simulink model "BCM_C1A_CombiSwitch_9"  (R2018b)
settings: Solver=FixedStepDiscrete  StartTime=0.0  StopTime=10.0  FixedStep=0.01  RelTol=1e-3
undefined symbols (not defined in the file or in its folder): TYP_CSW_INT_POSITION, TYP_EXT_LIGHTS, TYP_FRONT_WIPER, TYP_LIGHTING_CSW, TYP_REAR_WIPER, TYP_VEHICLE_STATE
libraries: Renault_Library x80, library_BCM x2
(part 3 of 3)

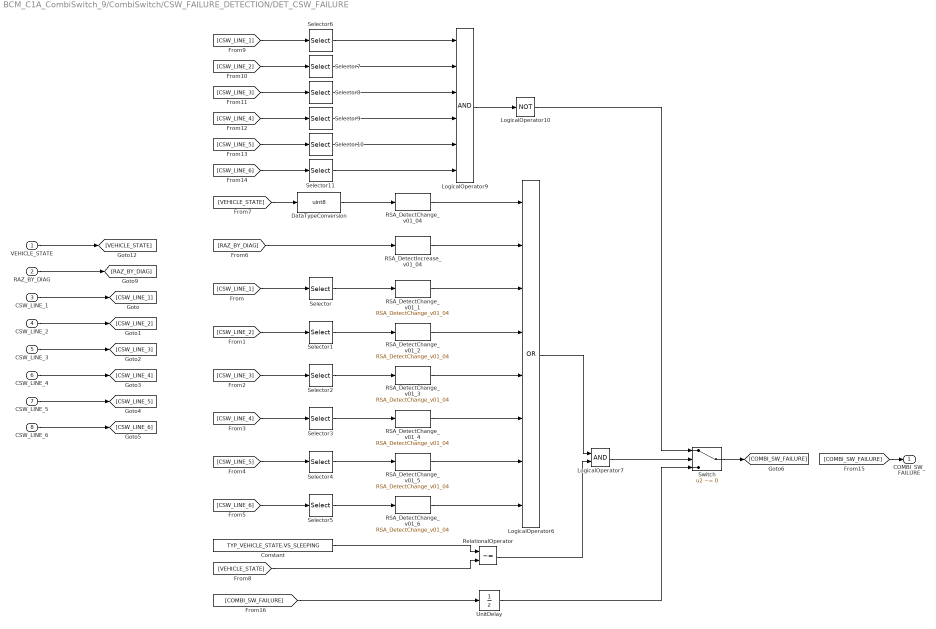
== system BCM_C1A_CombiSwitch_9/CombiSwitch/CSW_FAILURE_DETECTION/DET_CSW_FAILURE ==
  VEHICLE_STATE : Inport  OutDataTypeStr=Enum: TYP_VEHICLE_STATE
      settings: AttributesFormatString=Type : %<OutDataTypeStr>
  RAZ_BY_DIAG : Inport  Port=2  OutDataTypeStr=boolean
      settings: AttributesFormatString=Type : %<OutDataTypeStr>
  CSW_LINE_1 : Inport  Port=3  OutDataTypeStr=boolean  PortDimensions=6
      settings: AttributesFormatString=Type : %<OutDataTypeStr>
  CSW_LINE_2 : Inport  Port=4  OutDataTypeStr=boolean  PortDimensions=6
      settings: AttributesFormatString=Type : %<OutDataTypeStr>
  CSW_LINE_3 : Inport  Port=5  OutDataTypeStr=boolean  PortDimensions=6
      settings: AttributesFormatString=Type : %<OutDataTypeStr>
  CSW_LINE_4 : Inport  Port=6  OutDataTypeStr=boolean  PortDimensions=6
      settings: AttributesFormatString=Type : %<OutDataTypeStr>
  CSW_LINE_5 : Inport  Port=7  OutDataTypeStr=boolean  PortDimensions=6
      settings: AttributesFormatString=Type : %<OutDataTypeStr>
  CSW_LINE_6 : Inport  Port=8  OutDataTypeStr=boolean  PortDimensions=6
      settings: AttributesFormatString=Type : %<OutDataTypeStr>
  Constant : Constant  Value=TYP_VEHICLE_STATE.VS_SLEEPING  OutDataTypeStr=Enum: TYP_VEHICLE_STATE  SampleTime=-1
  DataTypeConversion : DataTypeConversion  OutDataTypeStr=uint8  RndMeth=Zero
      settings: AttributesFormatString=Saturation:%<SaturateOnIntegerOverflow>
  LogicalOperator10 : Logic  Operator=NOT  Inputs=1  OutDataTypeStr=boolean
  LogicalOperator6 : Logic  Operator=OR  Inputs=8  OutDataTypeStr=boolean
  LogicalOperator7 : Logic  OutDataTypeStr=boolean
  LogicalOperator9 : Logic  Inputs=6  OutDataTypeStr=boolean
  RSA_DetectChange_v01_04 : Renault_Library/Complex blocks/Logic & Bit Operations/RSA_DetectChange_v01_04  Tag=[LIB]  chkini=on  vinit=false
      settings: AttributesFormatString=%<MaskType> : Ver : 01.04\nCompare the Input with Initial Value = %<chkini>\nInitial Value : = %<vinit>
  RSA_DetectChange_v01_{1..6} (6 alike) : Renault_Library/Complex blocks/Logic & Bit Operations/RSA_DetectChange_v01_04  Tag=[LIB]  chkini=on  vinit=false
      settings: AttributesFormatString=%<MaskType> : Ver : 01.04\nCompare the Input with Initial Value = %<chkini>\nInitial Value : = %<vinit>
  RSA_DetectIncrease_v01_04 : Renault_Library/Complex blocks/Logic & Bit Operations/RSA_DetectIncrease_v01_04  Tag=[LIB]  chkini=on  vinit=false
      settings: AttributesFormatString=%<MaskType> : Ver : 01.04\nCompare the Input with Initial Value = %<chkini>\nInitial Value : = %<vinit>
  RelationalOperator : RelationalOperator  Operator=~=  OutDataTypeStr=boolean  RndMeth=Nearest  InputSameDT=on
  Selector : Selector  IndexMode=Zero-based  InputPortWidth=6  IndexOptions=Index vector (dialog)  Indices=[0]  OutputSizes=1
  Selector1 : Selector  IndexMode=Zero-based  InputPortWidth=6  IndexOptions=Index vector (dialog)  Indices=[1]  OutputSizes=1
  Selector10 : Selector  IndexMode=Zero-based  InputPortWidth=6  IndexOptions=Index vector (dialog)  Indices=[4]  OutputSizes=1
  Selector11 : Selector  IndexMode=Zero-based  InputPortWidth=6  IndexOptions=Index vector (dialog)  Indices=[5]  OutputSizes=1
  Selector2 : Selector  IndexMode=Zero-based  InputPortWidth=6  IndexOptions=Index vector (dialog)  Indices=[2]  OutputSizes=1
  Selector3 : Selector  IndexMode=Zero-based  InputPortWidth=6  IndexOptions=Index vector (dialog)  Indices=[3]  OutputSizes=1
  Selector4 : Selector  IndexMode=Zero-based  InputPortWidth=6  IndexOptions=Index vector (dialog)  Indices=[4]  OutputSizes=1
  Selector5 : Selector  IndexMode=Zero-based  InputPortWidth=6  IndexOptions=Index vector (dialog)  Indices=[5]  OutputSizes=1
  Selector6 : Selector  IndexMode=Zero-based  InputPortWidth=6  IndexOptions=Index vector (dialog)  Indices=[0]  OutputSizes=1
  Selector7 : Selector  IndexMode=Zero-based  InputPortWidth=6  IndexOptions=Index vector (dialog)  Indices=[1]  OutputSizes=1
  Selector8 : Selector  IndexMode=Zero-based  InputPortWidth=6  IndexOptions=Index vector (dialog)  Indices=[2]  OutputSizes=1
  Selector9 : Selector  IndexMode=Zero-based  InputPortWidth=6  IndexOptions=Index vector (dialog)  Indices=[3]  OutputSizes=1
  Switch : Switch  Criteria=u2 ~= 0  RndMeth=Zero  InputSameDT=on
      settings: AttributesFormatString=Criteria=%<Criteria>
  UnitDelay : UnitDelay  InitialCondition=false  SampleTime=-1
      settings: AttributesFormatString=IC = %<X0>
  COMBI_SW_FAILURE : Outport  OutDataTypeStr=boolean
      settings: AttributesFormatString=Type : %<OutDataTypeStr>\nInit :%<InitialOutput>
  wires:
  LogicalOperator9/1 -> LogicalOperator10/1
  Selector6/1 -> LogicalOperator9/1
  Selector8/1 -> LogicalOperator9/3
  Selector9/1 -> LogicalOperator9/4
  Selector10/1 -> LogicalOperator9/5
  Selector11/1 -> LogicalOperator9/6
  Selector7/1 -> LogicalOperator9/2
  [CSW_LINE_6] -> Selector11/1
  [CSW_LINE_5] -> Selector10/1
  [CSW_LINE_4] -> Selector9/1
  [CSW_LINE_3] -> Selector8/1
  [CSW_LINE_2] -> Selector7/1
  [CSW_LINE_1] -> Selector6/1
  LogicalOperator6/1 -> LogicalOperator7/1
  RelationalOperator/1 -> LogicalOperator7/2
  [VEHICLE_STATE] -> RelationalOperator/2
  Constant/1 -> RelationalOperator/1
  [RAZ_BY_DIAG] -> RSA_DetectIncrease_v01_04/1
  DataTypeConversion/1 -> RSA_DetectChange_v01_04/1
  [VEHICLE_STATE] -> DataTypeConversion/1
  Selector2/1 -> RSA_DetectChange_v01_3/1
  Selector3/1 -> RSA_DetectChange_v01_4/1
  Selector4/1 -> RSA_DetectChange_v01_5/1
  Selector5/1 -> RSA_DetectChange_v01_6/1
  Selector1/1 -> RSA_DetectChange_v01_2/1
  Selector/1 -> RSA_DetectChange_v01_1/1
  [CSW_LINE_6] -> Selector5/1
  [CSW_LINE_5] -> Selector4/1
  [CSW_LINE_4] -> Selector3/1
  [CSW_LINE_3] -> Selector2/1
  [CSW_LINE_2] -> Selector1/1
  [CSW_LINE_1] -> Selector/1
  CSW_LINE_6/1 -> [CSW_LINE_6]
  CSW_LINE_5/1 -> [CSW_LINE_5]
  CSW_LINE_4/1 -> [CSW_LINE_4]
  CSW_LINE_3/1 -> [CSW_LINE_3]
  CSW_LINE_2/1 -> [CSW_LINE_2]
  CSW_LINE_1/1 -> [CSW_LINE_1]
  RAZ_BY_DIAG/1 -> [RAZ_BY_DIAG]
  VEHICLE_STATE/1 -> [VEHICLE_STATE]
  LogicalOperator7/1 -> Switch/2
  LogicalOperator10/1 -> Switch/1
  Switch/1 -> [COMBI_SW_FAILURE]
  [COMBI_SW_FAILURE] -> UnitDelay/1
  [COMBI_SW_FAILURE] -> COMBI_SW_FAILURE/1
  UnitDelay/1 -> Switch/3
  RSA_DetectChange_v01_6/1 -> LogicalOperator6/8
  RSA_DetectChange_v01_5/1 -> LogicalOperator6/7
  RSA_DetectChange_v01_4/1 -> LogicalOperator6/6
  RSA_DetectChange_v01_3/1 -> LogicalOperator6/5
  RSA_DetectChange_v01_2/1 -> LogicalOperator6/4
  RSA_DetectChange_v01_1/1 -> LogicalOperator6/3
  RSA_DetectIncrease_v01_04/1 -> LogicalOperator6/2
  RSA_DetectChange_v01_04/1 -> LogicalOperator6/1

== system BCM_C1A_CombiSwitch_9/CombiSwitch/LIGHTING_FAILURE_DETECTION/DET_LIGHTING_FAILURE_3_POSITIONS ==
  VEHICLE_STATE : Inport  OutDataTypeStr=Enum: TYP_VEHICLE_STATE
      settings: AttributesFormatString=Type : %<OutDataTypeStr>
  RAZ_BY_DIAG : Inport  Port=2  OutDataTypeStr=boolean
      settings: AttributesFormatString=Type : %<OutDataTypeStr>
  CSW_LINE_2 : Inport  Port=3  OutDataTypeStr=boolean  PortDimensions=6
      settings: AttributesFormatString=Type : %<OutDataTypeStr>
  CSW_LINE_4 : Inport  Port=4  OutDataTypeStr=boolean  PortDimensions=6
      settings: AttributesFormatString=Type : %<OutDataTypeStr>
  Enable : EnablePort  StatesWhenEnabling=reset
      settings: AttributesFormatString=State : %<StatesWhenEnabling>
  Constant : Constant  Value=TYP_VEHICLE_STATE.VS_SLEEPING  OutDataTypeStr=Enum: TYP_VEHICLE_STATE  SampleTime=-1
  DataTypeConversion : DataTypeConversion  OutDataTypeStr=uint8  RndMeth=Zero
      settings: AttributesFormatString=Saturation:%<SaturateOnIntegerOverflow>
  LogicalOperator10 : Logic  Operator=NOT  Inputs=1  OutDataTypeStr=boolean
  LogicalOperator6 : Logic  Operator=OR  Inputs=5  OutDataTypeStr=boolean
  LogicalOperator7 : Logic  OutDataTypeStr=boolean
  LogicalOperator8 : Logic  Operator=OR  Inputs=3  OutDataTypeStr=boolean
  RSA_DetectChange_v01_04 : Renault_Library/Complex blocks/Logic & Bit Operations/RSA_DetectChange_v01_04  Tag=[LIB]  chkini=on  vinit=false
      settings: AttributesFormatString=%<MaskType> : Ver : 01.04\nCompare the Input with Initial Value = %<chkini>\nInitial Value : = %<vinit>
  RSA_DetectChange_v01_2 : Renault_Library/Complex blocks/Logic & Bit Operations/RSA_DetectChange_v01_04  Tag=[LIB]  chkini=on  vinit=false
      settings: AttributesFormatString=%<MaskType> : Ver : 01.04\nCompare the Input with Initial Value = %<chkini>\nInitial Value : = %<vinit>
  RSA_DetectChange_v01_4 : Renault_Library/Complex blocks/Logic & Bit Operations/RSA_DetectChange_v01_04  Tag=[LIB]  chkini=on  vinit=false
      settings: AttributesFormatString=%<MaskType> : Ver : 01.04\nCompare the Input with Initial Value = %<chkini>\nInitial Value : = %<vinit>
  RSA_DetectChange_v01_5 : Renault_Library/Complex blocks/Logic & Bit Operations/RSA_DetectChange_v01_04  Tag=[LIB]  chkini=on  vinit=false
      settings: AttributesFormatString=%<MaskType> : Ver : 01.04\nCompare the Input with Initial Value = %<chkini>\nInitial Value : = %<vinit>
  RSA_DetectIncrease_v01_04 : Renault_Library/Complex blocks/Logic & Bit Operations/RSA_DetectIncrease_v01_04  Tag=[LIB]  chkini=on  vinit=false
      settings: AttributesFormatString=%<MaskType> : Ver : 01.04\nCompare the Input with Initial Value = %<chkini>\nInitial Value : = %<vinit>
  RelationalOperator : RelationalOperator  Operator=~=  OutDataTypeStr=boolean  RndMeth=Nearest  InputSameDT=on
  Selector : Selector  IndexMode=Zero-based  InputPortWidth=6  IndexOptions=Index vector (dialog)  Indices=[2]  OutputSizes=1
  Selector{2..3,6..7} (4 alike) : Selector  IndexMode=Zero-based  InputPortWidth=6  IndexOptions=Index vector (dialog)  Indices=[4]  OutputSizes=1
  Selector4 : Selector  IndexMode=Zero-based  InputPortWidth=6  IndexOptions=Index vector (dialog)  Indices=[2]  OutputSizes=1
  Switch : Switch  Criteria=u2 ~= 0  RndMeth=Zero  InputSameDT=on
      settings: AttributesFormatString=Criteria=%<Criteria>
  UnitDelay : UnitDelay  InitialCondition=false  SampleTime=-1
      settings: AttributesFormatString=IC = %<X0>
  COMBI_SW_LIGHTING_FAILURE_3_POS : Outport  OutDataTypeStr=boolean  OutputWhenDisabled=reset  InitialOutput=false
      settings: AttributesFormatString=Type : %<OutDataTypeStr>\nInit :%<InitialOutput>
  wires:
  VEHICLE_STATE/1 -> [VEHICLE_STATE]
  RAZ_BY_DIAG/1 -> [RAZ_BY_DIAG]
  CSW_LINE_2/1 -> [CSW_LINE_2]
  CSW_LINE_4/1 -> [CSW_LINE_4]
  [CSW_LINE_2] -> Selector/1
  [CSW_LINE_2] -> Selector2/1
  [CSW_LINE_4] -> Selector3/1
  Selector/1 -> RSA_DetectChange_v01_2/1
  Selector3/1 -> RSA_DetectChange_v01_5/1
  Selector2/1 -> RSA_DetectChange_v01_4/1
  [VEHICLE_STATE] -> DataTypeConversion/1
  DataTypeConversion/1 -> RSA_DetectChange_v01_04/1
  [RAZ_BY_DIAG] -> RSA_DetectIncrease_v01_04/1
  RSA_DetectChange_v01_04/1 -> LogicalOperator6/1
  Constant/1 -> RelationalOperator/1
  [VEHICLE_STATE] -> RelationalOperator/2
  RelationalOperator/1 -> LogicalOperator7/2
  LogicalOperator6/1 -> LogicalOperator7/1
  LogicalOperator7/1 -> Switch/2
  Selector4/1 -> LogicalOperator8/1
  Selector6/1 -> LogicalOperator8/2
  LogicalOperator8/1 -> LogicalOperator10/1
  LogicalOperator10/1 -> Switch/1
  [COMBI_SW_LIGHTING_FAILURE_3_POS] -> UnitDelay/1
  UnitDelay/1 -> Switch/3
  [CSW_LINE_2] -> Selector4/1
  [CSW_LINE_2] -> Selector6/1
  [CSW_LINE_4] -> Selector7/1
  Selector7/1 -> LogicalOperator8/3
  Switch/1 -> COMBI_SW_LIGHTING_FAILURE_3_POS/1, [COMBI_SW_LIGHTING_FAILURE_3_POS]
  RSA_DetectIncrease_v01_04/1 -> LogicalOperator6/2
  RSA_DetectChange_v01_2/1 -> LogicalOperator6/3
  RSA_DetectChange_v01_4/1 -> LogicalOperator6/4
  RSA_DetectChange_v01_5/1 -> LogicalOperator6/5

== system BCM_C1A_CombiSwitch_9/CombiSwitch/LIGHTING_FAILURE_DETECTION/DET_LIGHTING_FAILURE_4_POSITIONS ==
  VEHICLE_STATE : Inport  OutDataTypeStr=Enum: TYP_VEHICLE_STATE
      settings: AttributesFormatString=Type : %<OutDataTypeStr>
  RAZ_BY_DIAG : Inport  Port=2  OutDataTypeStr=boolean
      settings: AttributesFormatString=Type : %<OutDataTypeStr>
  CSW_LINE_2 : Inport  Port=3  OutDataTypeStr=boolean  PortDimensions=6
      settings: AttributesFormatString=Type : %<OutDataTypeStr>
  CSW_LINE_4 : Inport  Port=4  OutDataTypeStr=boolean  PortDimensions=6
      settings: AttributesFormatString=Type : %<OutDataTypeStr>
  Enable : EnablePort  StatesWhenEnabling=reset
      settings: AttributesFormatString=State : %<StatesWhenEnabling>
  Constant : Constant  Value=TYP_VEHICLE_STATE.VS_SLEEPING  OutDataTypeStr=Enum: TYP_VEHICLE_STATE  SampleTime=-1
  DataTypeConversion : DataTypeConversion  OutDataTypeStr=uint8  RndMeth=Zero
      settings: AttributesFormatString=Saturation:%<SaturateOnIntegerOverflow>
  LogicalOperator10 : Logic  Operator=NOT  Inputs=1  OutDataTypeStr=boolean
  LogicalOperator6 : Logic  Operator=OR  Inputs=6  OutDataTypeStr=boolean
  LogicalOperator7 : Logic  OutDataTypeStr=boolean
  LogicalOperator8 : Logic  Operator=OR  Inputs=4  OutDataTypeStr=boolean
  RSA_DetectChange_v01_04 : Renault_Library/Complex blocks/Logic & Bit Operations/RSA_DetectChange_v01_04  Tag=[LIB]  chkini=on  vinit=false
      settings: AttributesFormatString=%<MaskType> : Ver : 01.04\nCompare the Input with Initial Value = %<chkini>\nInitial Value : = %<vinit>
  RSA_DetectChange_v01_{2..5} (4 alike) : Renault_Library/Complex blocks/Logic & Bit Operations/RSA_DetectChange_v01_04  Tag=[LIB]  chkini=on  vinit=false
      settings: AttributesFormatString=%<MaskType> : Ver : 01.04\nCompare the Input with Initial Value = %<chkini>\nInitial Value : = %<vinit>
  RSA_DetectIncrease_v01_04 : Renault_Library/Complex blocks/Logic & Bit Operations/RSA_DetectIncrease_v01_04  Tag=[LIB]  chkini=on  vinit=false
      settings: AttributesFormatString=%<MaskType> : Ver : 01.04\nCompare the Input with Initial Value = %<chkini>\nInitial Value : = %<vinit>
  RelationalOperator : RelationalOperator  Operator=~=  OutDataTypeStr=boolean  RndMeth=Nearest  InputSameDT=on
  Selector : Selector  IndexMode=Zero-based  InputPortWidth=6  IndexOptions=Index vector (dialog)  Indices=[2]  OutputSizes=1
  Selector1 : Selector  IndexMode=Zero-based  InputPortWidth=6  IndexOptions=Index vector (dialog)  Indices=[3]  OutputSizes=1
  Selector{2..3,6..7} (4 alike) : Selector  IndexMode=Zero-based  InputPortWidth=6  IndexOptions=Index vector (dialog)  Indices=[4]  OutputSizes=1
  Selector4 : Selector  IndexMode=Zero-based  InputPortWidth=6  IndexOptions=Index vector (dialog)  Indices=[2]  OutputSizes=1
  Selector5 : Selector  IndexMode=Zero-based  InputPortWidth=6  IndexOptions=Index vector (dialog)  Indices=[3]  OutputSizes=1
  Switch : Switch  Criteria=u2 ~= 0  RndMeth=Zero  InputSameDT=on
      settings: AttributesFormatString=Criteria=%<Criteria>
  UnitDelay : UnitDelay  InitialCondition=false  SampleTime=-1
      settings: AttributesFormatString=IC = %<X0>
  COMBI_SW_LIGHTING_FAILURE_4_POS : Outport  OutDataTypeStr=boolean  OutputWhenDisabled=reset  InitialOutput=false
      settings: AttributesFormatString=Type : %<OutDataTypeStr>\nInit :%<InitialOutput>
  wires:
  Switch/1 -> [COMBI_SW_LIGHTING_FAILURE_4_POS], COMBI_SW_LIGHTING_FAILURE_4_POS/1
  [CSW_LINE_4] -> Selector7/1
  [CSW_LINE_2] -> Selector6/1
  [CSW_LINE_2] -> Selector5/1
  [CSW_LINE_2] -> Selector4/1
  UnitDelay/1 -> Switch/3
  [COMBI_SW_LIGHTING_FAILURE_4_POS] -> UnitDelay/1
  LogicalOperator10/1 -> Switch/1
  LogicalOperator8/1 -> LogicalOperator10/1
  Selector5/1 -> LogicalOperator8/2
  Selector4/1 -> LogicalOperator8/1
  LogicalOperator7/1 -> Switch/2
  LogicalOperator6/1 -> LogicalOperator7/1
  RelationalOperator/1 -> LogicalOperator7/2
  [VEHICLE_STATE] -> RelationalOperator/2
  Constant/1 -> RelationalOperator/1
  RSA_DetectChange_v01_04/1 -> LogicalOperator6/1
  RSA_DetectIncrease_v01_04/1 -> LogicalOperator6/2
  [RAZ_BY_DIAG] -> RSA_DetectIncrease_v01_04/1
  DataTypeConversion/1 -> RSA_DetectChange_v01_04/1
  [VEHICLE_STATE] -> DataTypeConversion/1
  RSA_DetectChange_v01_5/1 -> LogicalOperator6/6
  RSA_DetectChange_v01_4/1 -> LogicalOperator6/5
  RSA_DetectChange_v01_3/1 -> LogicalOperator6/4
  RSA_DetectChange_v01_2/1 -> LogicalOperator6/3
  Selector2/1 -> RSA_DetectChange_v01_4/1
  Selector3/1 -> RSA_DetectChange_v01_5/1
  Selector1/1 -> RSA_DetectChange_v01_3/1
  Selector/1 -> RSA_DetectChange_v01_2/1
  [CSW_LINE_4] -> Selector3/1
  [CSW_LINE_2] -> Selector2/1
  [CSW_LINE_2] -> Selector1/1
  [CSW_LINE_2] -> Selector/1
  CSW_LINE_4/1 -> [CSW_LINE_4]
  CSW_LINE_2/1 -> [CSW_LINE_2]
  RAZ_BY_DIAG/1 -> [RAZ_BY_DIAG]
  VEHICLE_STATE/1 -> [VEHICLE_STATE]
  Selector6/1 -> LogicalOperator8/3
  Selector7/1 -> LogicalOperator8/4

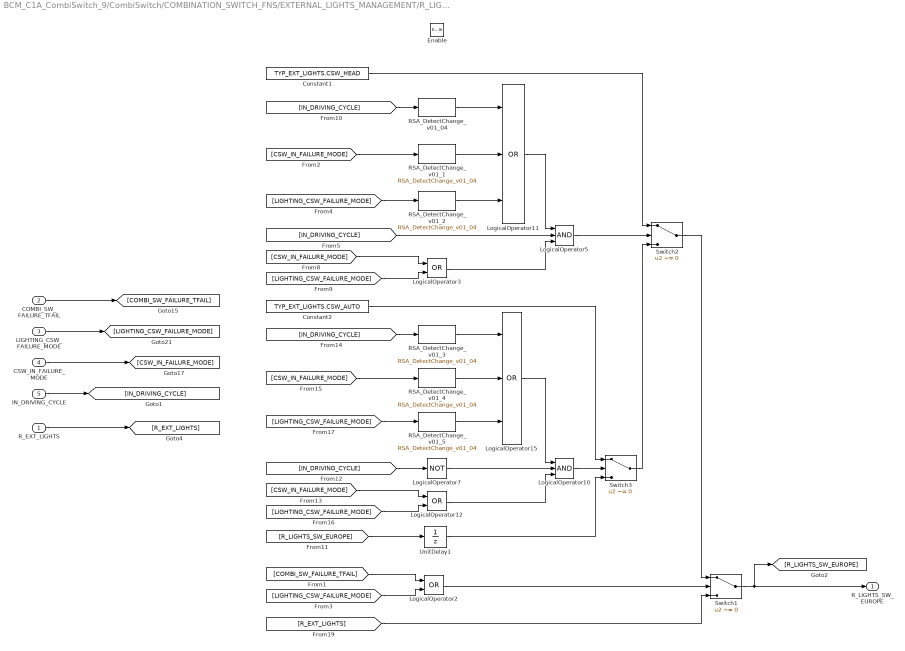
== system BCM_C1A_CombiSwitch_9/CombiSwitch/COMBINATION_SWITCH_FNS/EXTERNAL_LIGHTS_MANAGEMENT/R_LIGHT_SW_EUROPE ==
  R_EXT_LIGHTS : Inport  OutDataTypeStr=Enum: TYP_EXT_LIGHTS
      settings: AttributesFormatString=Type : %<OutDataTypeStr>
  COMBI_SW_FAILURE_TFAIL : Inport  Port=2  OutDataTypeStr=boolean
      settings: AttributesFormatString=Type : %<OutDataTypeStr>
  LIGHTING_CSW_FAILURE_MODE : Inport  Port=3  OutDataTypeStr=boolean
      settings: AttributesFormatString=Type : %<OutDataTypeStr>
  CSW_IN_FAILURE_MODE : Inport  Port=4  OutDataTypeStr=boolean
      settings: AttributesFormatString=Type : %<OutDataTypeStr>
  IN_DRIVING_CYCLE : Inport  Port=5  OutDataTypeStr=boolean
      settings: AttributesFormatString=Type : %<OutDataTypeStr>
  Enable : EnablePort  StatesWhenEnabling=reset
      settings: AttributesFormatString=State : %<StatesWhenEnabling>
  Constant1 : Constant  Value=TYP_EXT_LIGHTS.CSW_HEAD  OutDataTypeStr=Enum: TYP_EXT_LIGHTS  SampleTime=-1
  Constant2 : Constant  Value=TYP_EXT_LIGHTS.CSW_AUTO  OutDataTypeStr=Enum: TYP_EXT_LIGHTS  SampleTime=-1
  LogicalOperator10 : Logic  Inputs=3  OutDataTypeStr=boolean
  LogicalOperator11 : Logic  Operator=OR  Inputs=3  OutDataTypeStr=boolean
  LogicalOperator12 : Logic  Operator=OR  OutDataTypeStr=boolean
  LogicalOperator15 : Logic  Operator=OR  Inputs=3  OutDataTypeStr=boolean
  LogicalOperator2 : Logic  Operator=OR  OutDataTypeStr=boolean
  LogicalOperator3 : Logic  Operator=OR  OutDataTypeStr=boolean
  LogicalOperator5 : Logic  Inputs=3  OutDataTypeStr=boolean
  LogicalOperator7 : Logic  Operator=NOT  Inputs=1  OutDataTypeStr=boolean
  RSA_DetectChange_v01_04 : Renault_Library/Complex blocks/Logic & Bit Operations/RSA_DetectChange_v01_04  Tag=[LIB]  chkini=on  vinit=false
      settings: AttributesFormatString=%<MaskType> : Ver : 01.04\nCompare the Input with Initial Value = %<chkini>\nInitial Value : = %<vinit>
  RSA_DetectChange_v01_{1..5} (5 alike) : Renault_Library/Complex blocks/Logic & Bit Operations/RSA_DetectChange_v01_04  Tag=[LIB]  chkini=on  vinit=false
      settings: AttributesFormatString=%<MaskType> : Ver : 01.04\nCompare the Input with Initial Value = %<chkini>\nInitial Value : = %<vinit>
  Switch1 : Switch  Criteria=u2 ~= 0  RndMeth=Zero  InputSameDT=on
      settings: AttributesFormatString=Criteria=%<Criteria>
  Switch2 : Switch  Criteria=u2 ~= 0  RndMeth=Zero  InputSameDT=on
      settings: AttributesFormatString=Criteria=%<Criteria>
  Switch3 : Switch  Criteria=u2 ~= 0  RndMeth=Zero  InputSameDT=on
      settings: AttributesFormatString=Criteria=%<Criteria>
  UnitDelay1 : UnitDelay  InitialCondition=TYP_EXT_LIGHTS.CSW_AUTO  SampleTime=-1
      settings: AttributesFormatString=IC = %<X0>
  R_LIGHTS_SW_EUROPE : Outport  OutDataTypeStr=Enum: TYP_EXT_LIGHTS  OutputWhenDisabled=reset  InitialOutput=TYP_EXT_LIGHTS.CSW_AUTO
      settings: AttributesFormatString=Type : %<OutDataTypeStr>\nInit :%<InitialOutput>
  wires:
  RSA_DetectChange_v01_4/1 -> LogicalOperator15/2
  Constant1/1 -> Switch2/1
  LogicalOperator2/1 -> Switch1/2
  [CSW_IN_FAILURE_MODE] -> LogicalOperator3/1
  UnitDelay1/1 -> Switch3/3
  LogicalOperator11/1 -> LogicalOperator5/1
  LogicalOperator12/1 -> LogicalOperator10/3
  RSA_DetectChange_v01_1/1 -> LogicalOperator11/2
  Switch3/1 -> Switch2/3
  LogicalOperator5/1 -> Switch2/2
  Constant2/1 -> Switch3/1
  [LIGHTING_CSW_FAILURE_MODE] -> RSA_DetectChange_v01_2/1
  [LIGHTING_CSW_FAILURE_MODE] -> LogicalOperator2/2
  IN_DRIVING_CYCLE/1 -> [IN_DRIVING_CYCLE]
  CSW_IN_FAILURE_MODE/1 -> [CSW_IN_FAILURE_MODE]
  R_EXT_LIGHTS/1 -> [R_EXT_LIGHTS]
  LogicalOperator10/1 -> Switch3/2
  Switch1/1 -> R_LIGHTS_SW_EUROPE/1, [R_LIGHTS_SW_EUROPE]
  Switch2/1 -> Switch1/1
  [CSW_IN_FAILURE_MODE] -> RSA_DetectChange_v01_4/1
  [CSW_IN_FAILURE_MODE] -> RSA_DetectChange_v01_1/1
  COMBI_SW_FAILURE_TFAIL/1 -> [COMBI_SW_FAILURE_TFAIL]
  RSA_DetectChange_v01_04/1 -> LogicalOperator11/1
  [IN_DRIVING_CYCLE] -> RSA_DetectChange_v01_3/1
  RSA_DetectChange_v01_3/1 -> LogicalOperator15/1
  [COMBI_SW_FAILURE_TFAIL] -> LogicalOperator2/1
  [IN_DRIVING_CYCLE] -> RSA_DetectChange_v01_04/1
  [R_LIGHTS_SW_EUROPE] -> UnitDelay1/1
  [IN_DRIVING_CYCLE] -> LogicalOperator7/1
  [LIGHTING_CSW_FAILURE_MODE] -> LogicalOperator12/2
  LogicalOperator7/1 -> LogicalOperator10/2
  [R_EXT_LIGHTS] -> Switch1/3
  LIGHTING_CSW_FAILURE_MODE/1 -> [LIGHTING_CSW_FAILURE_MODE]
  RSA_DetectChange_v01_2/1 -> LogicalOperator11/3
  [CSW_IN_FAILURE_MODE] -> LogicalOperator12/1
  [LIGHTING_CSW_FAILURE_MODE] -> RSA_DetectChange_v01_5/1
  [LIGHTING_CSW_FAILURE_MODE] -> LogicalOperator3/2
  [IN_DRIVING_CYCLE] -> LogicalOperator5/2
  LogicalOperator3/1 -> LogicalOperator5/3
  LogicalOperator15/1 -> LogicalOperator10/1
  RSA_DetectChange_v01_5/1 -> LogicalOperator15/3

== system BCM_C1A_CombiSwitch_9/CombiSwitch/COMBINATION_SWITCH_FNS/EXTERNAL_LIGHTS_MANAGEMENT/R_LIGHT_SW_WORLD ==
  R_EXT_LIGHTS : Inport  OutDataTypeStr=Enum: TYP_EXT_LIGHTS
      settings: AttributesFormatString=Type : %<OutDataTypeStr>
  COMBI_SW_FAILURE_TFAIL : Inport  Port=2  OutDataTypeStr=boolean
      settings: AttributesFormatString=Type : %<OutDataTypeStr>
  LIGHTING_CSW_FAILURE_MODE : Inport  Port=3  OutDataTypeStr=boolean
      settings: AttributesFormatString=Type : %<OutDataTypeStr>
  CSW_IN_FAILURE_MODE : Inport  Port=4  OutDataTypeStr=boolean
      settings: AttributesFormatString=Type : %<OutDataTypeStr>
  IN_DRIVING_CYCLE : Inport  Port=5  OutDataTypeStr=boolean
      settings: AttributesFormatString=Type : %<OutDataTypeStr>
  Enable : EnablePort  StatesWhenEnabling=reset
      settings: AttributesFormatString=State : %<StatesWhenEnabling>
  Constant1 : Constant  Value=TYP_EXT_LIGHTS.CSW_HEAD  OutDataTypeStr=Enum: TYP_EXT_LIGHTS  SampleTime=-1
  Constant2 : Constant  Value=TYP_EXT_LIGHTS.CSW_OFF_EL  OutDataTypeStr=Enum: TYP_EXT_LIGHTS  SampleTime=-1
  LogicalOperator10 : Logic  Inputs=3  OutDataTypeStr=boolean
  LogicalOperator11 : Logic  Operator=OR  Inputs=3  OutDataTypeStr=boolean
  LogicalOperator12 : Logic  Operator=OR  OutDataTypeStr=boolean
  LogicalOperator2 : Logic  Operator=OR  OutDataTypeStr=boolean
  LogicalOperator3 : Logic  Operator=OR  OutDataTypeStr=boolean
  LogicalOperator5 : Logic  Inputs=3  OutDataTypeStr=boolean
  LogicalOperator7 : Logic  Operator=NOT  Inputs=1  OutDataTypeStr=boolean
  LogicalOperator9 : Logic  Operator=OR  Inputs=3  OutDataTypeStr=boolean
  RSA_DetectChange_v01_04 : Renault_Library/Complex blocks/Logic & Bit Operations/RSA_DetectChange_v01_04  Tag=[LIB]  chkini=on  vinit=false
      settings: AttributesFormatString=%<MaskType> : Ver : 01.04\nCompare the Input with Initial Value = %<chkini>\nInitial Value : = %<vinit>
  RSA_DetectChange_v01_{1..5} (5 alike) : Renault_Library/Complex blocks/Logic & Bit Operations/RSA_DetectChange_v01_04  Tag=[LIB]  chkini=on  vinit=false
      settings: AttributesFormatString=%<MaskType> : Ver : 01.04\nCompare the Input with Initial Value = %<chkini>\nInitial Value : = %<vinit>
  Switch1 : Switch  Criteria=u2 ~= 0  RndMeth=Zero  InputSameDT=on
      settings: AttributesFormatString=Criteria=%<Criteria>
  Switch2 : Switch  Criteria=u2 ~= 0  RndMeth=Zero  InputSameDT=on
      settings: AttributesFormatString=Criteria=%<Criteria>
  Switch3 : Switch  Criteria=u2 ~= 0  RndMeth=Zero  InputSameDT=on
      settings: AttributesFormatString=Criteria=%<Criteria>
  UnitDelay1 : UnitDelay  InitialCondition=TYP_EXT_LIGHTS.CSW_OFF_EL  SampleTime=-1
      settings: AttributesFormatString=IC = %<X0>
  R_LIGHTS_SW_WORLD : Outport  OutDataTypeStr=Enum: TYP_EXT_LIGHTS  OutputWhenDisabled=reset  InitialOutput=TYP_EXT_LIGHTS.CSW_OFF_EL
      settings: AttributesFormatString=Type : %<OutDataTypeStr>\nInit :%<InitialOutput>
  wires:
  LogicalOperator9/1 -> LogicalOperator10/1
  LogicalOperator3/1 -> LogicalOperator5/3
  [LIGHTING_CSW_FAILURE_MODE] -> LogicalOperator3/2
  [LIGHTING_CSW_FAILURE_MODE] -> RSA_DetectChange_v01_5/1
  [CSW_IN_FAILURE_MODE] -> LogicalOperator12/1
  LIGHTING_CSW_FAILURE_MODE/1 -> [LIGHTING_CSW_FAILURE_MODE]
  [R_EXT_LIGHTS] -> Switch1/3
  LogicalOperator7/1 -> LogicalOperator10/2
  [LIGHTING_CSW_FAILURE_MODE] -> LogicalOperator12/2
  [IN_DRIVING_CYCLE] -> LogicalOperator7/1
  [R_LIGHTS_SW_WORLD] -> UnitDelay1/1
  [IN_DRIVING_CYCLE] -> RSA_DetectChange_v01_04/1
  [COMBI_SW_FAILURE_TFAIL] -> LogicalOperator2/1
  RSA_DetectChange_v01_3/1 -> LogicalOperator9/1
  [IN_DRIVING_CYCLE] -> RSA_DetectChange_v01_3/1
  RSA_DetectChange_v01_04/1 -> LogicalOperator11/1
  COMBI_SW_FAILURE_TFAIL/1 -> [COMBI_SW_FAILURE_TFAIL]
  [CSW_IN_FAILURE_MODE] -> RSA_DetectChange_v01_1/1
  [CSW_IN_FAILURE_MODE] -> RSA_DetectChange_v01_4/1
  Switch2/1 -> Switch1/1
  Switch1/1 -> R_LIGHTS_SW_WORLD/1, [R_LIGHTS_SW_WORLD]
  LogicalOperator10/1 -> Switch3/2
  R_EXT_LIGHTS/1 -> [R_EXT_LIGHTS]
  CSW_IN_FAILURE_MODE/1 -> [CSW_IN_FAILURE_MODE]
  IN_DRIVING_CYCLE/1 -> [IN_DRIVING_CYCLE]
  [IN_DRIVING_CYCLE] -> LogicalOperator5/2
  [LIGHTING_CSW_FAILURE_MODE] -> LogicalOperator2/2
  [LIGHTING_CSW_FAILURE_MODE] -> RSA_DetectChange_v01_2/1
  Constant2/1 -> Switch3/1
  LogicalOperator5/1 -> Switch2/2
  Switch3/1 -> Switch2/3
  RSA_DetectChange_v01_1/1 -> LogicalOperator11/2
  LogicalOperator12/1 -> LogicalOperator10/3
  LogicalOperator11/1 -> LogicalOperator5/1
  UnitDelay1/1 -> Switch3/3
  [CSW_IN_FAILURE_MODE] -> LogicalOperator3/1
  RSA_DetectChange_v01_5/1 -> LogicalOperator9/3
  LogicalOperator2/1 -> Switch1/2
  Constant1/1 -> Switch2/1
  RSA_DetectChange_v01_4/1 -> LogicalOperator9/2
  RSA_DetectChange_v01_2/1 -> LogicalOperator11/3

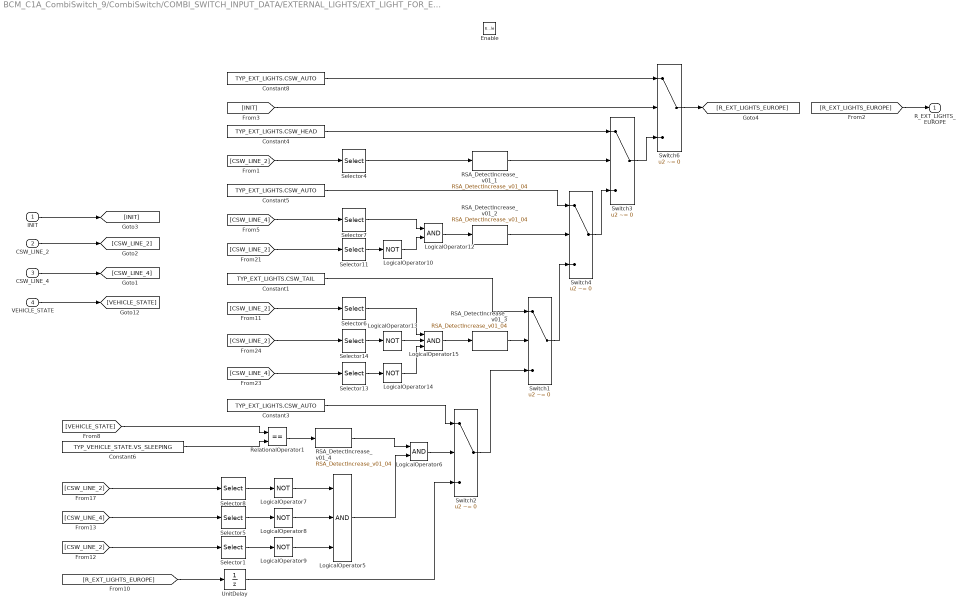
== system BCM_C1A_CombiSwitch_9/CombiSwitch/COMBI_SWITCH_INPUT_DATA/EXTERNAL_LIGHTS/EXT_LIGHT_FOR_EUROPE ==
  INIT : Inport  OutDataTypeStr=boolean
      settings: AttributesFormatString=Type : %<OutDataTypeStr>
  CSW_LINE_2 : Inport  Port=2  OutDataTypeStr=boolean  PortDimensions=6
      settings: AttributesFormatString=Type : %<OutDataTypeStr>
  CSW_LINE_4 : Inport  Port=3  OutDataTypeStr=boolean  PortDimensions=6
      settings: AttributesFormatString=Type : %<OutDataTypeStr>
  VEHICLE_STATE : Inport  Port=4  OutDataTypeStr=Enum: TYP_VEHICLE_STATE
      settings: AttributesFormatString=Type : %<OutDataTypeStr>
  Enable : EnablePort  StatesWhenEnabling=reset
      settings: AttributesFormatString=State : %<StatesWhenEnabling>
  Constant1 : Constant  Value=TYP_EXT_LIGHTS.CSW_TAIL  OutDataTypeStr=Enum: TYP_EXT_LIGHTS  SampleTime=-1
  Constant3 : Constant  Value=TYP_EXT_LIGHTS.CSW_AUTO  OutDataTypeStr=Enum: TYP_EXT_LIGHTS  SampleTime=-1
  Constant4 : Constant  Value=TYP_EXT_LIGHTS.CSW_HEAD  OutDataTypeStr=Enum: TYP_EXT_LIGHTS  SampleTime=-1
  Constant5 : Constant  Value=TYP_EXT_LIGHTS.CSW_AUTO  OutDataTypeStr=Enum: TYP_EXT_LIGHTS  SampleTime=-1
  Constant6 : Constant  Value=TYP_VEHICLE_STATE.VS_SLEEPING  OutDataTypeStr=Enum: TYP_VEHICLE_STATE  SampleTime=-1
  Constant8 : Constant  Value=TYP_EXT_LIGHTS.CSW_AUTO  OutDataTypeStr=Enum: TYP_EXT_LIGHTS  SampleTime=-1
  LogicalOperator{7..10,13..14} (6 alike) : Logic  Operator=NOT  OutDataTypeStr=boolean
  LogicalOperator12 : Logic  OutDataTypeStr=boolean
  LogicalOperator15 : Logic  Inputs=3  OutDataTypeStr=boolean
  LogicalOperator5 : Logic  Inputs=3  OutDataTypeStr=boolean
  LogicalOperator6 : Logic  OutDataTypeStr=boolean
  RSA_DetectIncrease_v01_{1..4} (4 alike) : Renault_Library/Complex blocks/Logic & Bit Operations/RSA_DetectIncrease_v01_04  Tag=[LIB]  chkini=off  vinit=false
      settings: AttributesFormatString=%<MaskType> : Ver : 01.04\nCompare the Input with Initial Value = %<chkini>\nInitial Value : = %<vinit>
  RelationalOperator1 : RelationalOperator  Operator===  OutDataTypeStr=boolean  RndMeth=Nearest  InputSameDT=on
  Selector{1,5..7,13} (5 alike) : Selector  IndexMode=Zero-based  InputPortWidth=6  IndexOptions=Index vector (dialog)  Indices=[4]  OutputSizes=1
  Selector{4,8,11,14} (4 alike) : Selector  IndexMode=Zero-based  InputPortWidth=6  IndexOptions=Index vector (dialog)  Indices=[2]  OutputSizes=1
  Switch{1..4,6} (5 alike) : Switch  Criteria=u2 ~= 0  RndMeth=Zero  InputSameDT=on
      settings: AttributesFormatString=Criteria=%<Criteria>
  UnitDelay : UnitDelay  InitialCondition=TYP_EXT_LIGHTS.CSW_OFF_EL  SampleTime=-1
      settings: AttributesFormatString=IC = %<X0>
  R_EXT_LIGHTS_EUROPE : Outport  OutDataTypeStr=Enum: TYP_EXT_LIGHTS  OutputWhenDisabled=reset  InitialOutput=TYP_EXT_LIGHTS.CSW_AUTO
      settings: AttributesFormatString=Type : %<OutDataTypeStr>\nInit :%<InitialOutput>
  wires:
  CSW_LINE_4/1 -> [CSW_LINE_4]
  VEHICLE_STATE/1 -> [VEHICLE_STATE]
  INIT/1 -> [INIT]
  CSW_LINE_2/1 -> [CSW_LINE_2]
  [INIT] -> Switch6/2
  Switch6/1 -> [R_EXT_LIGHTS_EUROPE]
  Constant4/1 -> Switch3/1
  Switch3/1 -> Switch6/3
  Constant8/1 -> Switch6/1
  [R_EXT_LIGHTS_EUROPE] -> R_EXT_LIGHTS_EUROPE/1
  [R_EXT_LIGHTS_EUROPE] -> UnitDelay/1
  Switch4/1 -> Switch3/3
  Switch1/1 -> Switch4/3
  [CSW_LINE_2] -> Selector4/1
  [CSW_LINE_2] -> Selector6/1
  [CSW_LINE_4] -> Selector7/1
  Selector6/1 -> LogicalOperator15/1
  Constant1/1 -> Switch1/1
  Selector7/1 -> LogicalOperator12/1
  Constant5/1 -> Switch4/1
  Selector4/1 -> RSA_DetectIncrease_v01_1/1
  LogicalOperator12/1 -> RSA_DetectIncrease_v01_2/1
  LogicalOperator15/1 -> RSA_DetectIncrease_v01_3/1
  Constant6/1 -> RelationalOperator1/2
  [VEHICLE_STATE] -> RelationalOperator1/1
  RelationalOperator1/1 -> RSA_DetectIncrease_v01_4/1
  [CSW_LINE_2] -> Selector1/1
  Selector1/1 -> LogicalOperator9/1
  [CSW_LINE_4] -> Selector5/1
  Selector5/1 -> LogicalOperator8/1
  [CSW_LINE_2] -> Selector8/1
  Selector8/1 -> LogicalOperator7/1
  LogicalOperator5/1 -> LogicalOperator6/2
  RSA_DetectIncrease_v01_4/1 -> LogicalOperator6/1
  LogicalOperator6/1 -> Switch2/2
  Switch2/1 -> Switch1/3
  Constant3/1 -> Switch2/1
  UnitDelay/1 -> Switch2/3
  [CSW_LINE_2] -> Selector11/1
  Selector11/1 -> LogicalOperator10/1
  LogicalOperator10/1 -> LogicalOperator12/2
  [CSW_LINE_4] -> Selector13/1
  [CSW_LINE_2] -> Selector14/1
  Selector14/1 -> LogicalOperator13/1
  Selector13/1 -> LogicalOperator14/1
  LogicalOperator13/1 -> LogicalOperator15/2
  LogicalOperator14/1 -> LogicalOperator15/3
  RSA_DetectIncrease_v01_1/1 -> Switch3/2
  RSA_DetectIncrease_v01_2/1 -> Switch4/2
  RSA_DetectIncrease_v01_3/1 -> Switch1/2
  LogicalOperator7/1 -> LogicalOperator5/1
  LogicalOperator8/1 -> LogicalOperator5/2
  LogicalOperator9/1 -> LogicalOperator5/3

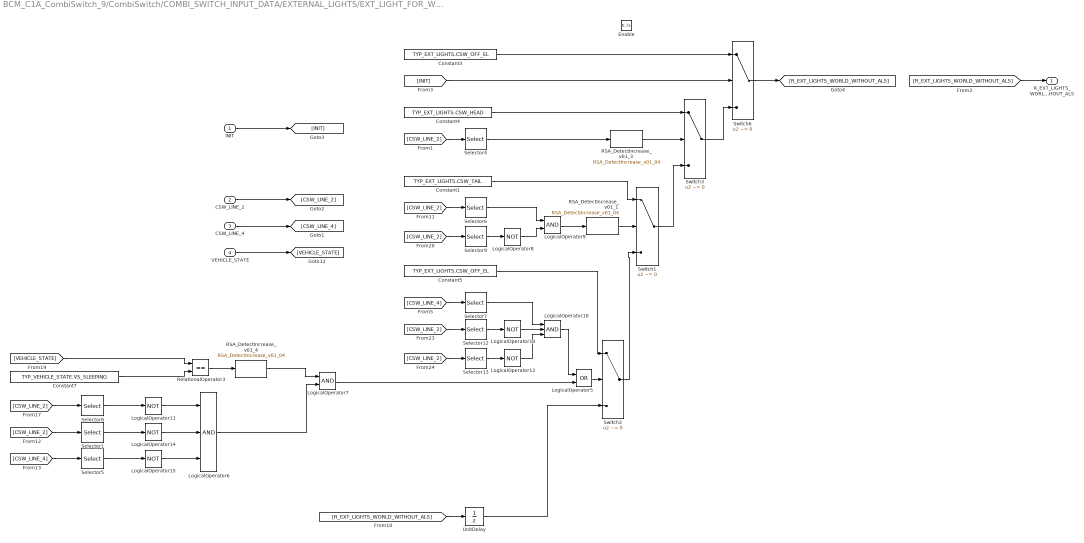
== system BCM_C1A_CombiSwitch_9/CombiSwitch/COMBI_SWITCH_INPUT_DATA/EXTERNAL_LIGHTS/EXT_LIGHT_FOR_WORLD_WITHOUT_ALS ==
  INIT : Inport  OutDataTypeStr=boolean
      settings: AttributesFormatString=Type : %<OutDataTypeStr>
  CSW_LINE_2 : Inport  Port=2  OutDataTypeStr=boolean  PortDimensions=6
      settings: AttributesFormatString=Type : %<OutDataTypeStr>
  CSW_LINE_4 : Inport  Port=3  OutDataTypeStr=boolean  PortDimensions=6
      settings: AttributesFormatString=Type : %<OutDataTypeStr>
  VEHICLE_STATE : Inport  Port=4  OutDataTypeStr=Enum: TYP_VEHICLE_STATE
      settings: AttributesFormatString=Type : %<OutDataTypeStr>
  Enable : EnablePort  StatesWhenEnabling=reset
      settings: AttributesFormatString=State : %<StatesWhenEnabling>
  Constant1 : Constant  Value=TYP_EXT_LIGHTS.CSW_TAIL  OutDataTypeStr=Enum: TYP_EXT_LIGHTS  SampleTime=-1
  Constant3 : Constant  Value=TYP_EXT_LIGHTS.CSW_OFF_EL  OutDataTypeStr=Enum: TYP_EXT_LIGHTS  SampleTime=-1
  Constant4 : Constant  Value=TYP_EXT_LIGHTS.CSW_HEAD  OutDataTypeStr=Enum: TYP_EXT_LIGHTS  SampleTime=-1
  Constant5 : Constant  Value=TYP_EXT_LIGHTS.CSW_OFF_EL  OutDataTypeStr=Enum: TYP_EXT_LIGHTS  SampleTime=-1
  Constant7 : Constant  Value=TYP_VEHICLE_STATE.VS_SLEEPING  OutDataTypeStr=Enum: TYP_VEHICLE_STATE  SampleTime=-1
  LogicalOperator10 : Logic  Inputs=3  OutDataTypeStr=boolean
  LogicalOperator{8,11..15} (6 alike) : Logic  Operator=NOT  OutDataTypeStr=boolean
  LogicalOperator5 : Logic  Operator=OR  OutDataTypeStr=boolean
  LogicalOperator6 : Logic  Inputs=3  OutDataTypeStr=boolean
  LogicalOperator7 : Logic  OutDataTypeStr=boolean
  LogicalOperator9 : Logic  OutDataTypeStr=boolean
  RSA_DetectIncrease_v01_1 : Renault_Library/Complex blocks/Logic & Bit Operations/RSA_DetectIncrease_v01_04  Tag=[LIB]  chkini=off  vinit=false
      settings: AttributesFormatString=%<MaskType> : Ver : 01.04\nCompare the Input with Initial Value = %<chkini>\nInitial Value : = %<vinit>
  RSA_DetectIncrease_v01_3 : Renault_Library/Complex blocks/Logic & Bit Operations/RSA_DetectIncrease_v01_04  Tag=[LIB]  chkini=off  vinit=false
      settings: AttributesFormatString=%<MaskType> : Ver : 01.04\nCompare the Input with Initial Value = %<chkini>\nInitial Value : = %<vinit>
  RSA_DetectIncrease_v01_4 : Renault_Library/Complex blocks/Logic & Bit Operations/RSA_DetectIncrease_v01_04  Tag=[LIB]  chkini=off  vinit=false
      settings: AttributesFormatString=%<MaskType> : Ver : 01.04\nCompare the Input with Initial Value = %<chkini>\nInitial Value : = %<vinit>
  RelationalOperator3 : RelationalOperator  Operator===  OutDataTypeStr=boolean  RndMeth=Nearest  InputSameDT=on
  Selector{1,5..7,12} (5 alike) : Selector  IndexMode=Zero-based  InputPortWidth=6  IndexOptions=Index vector (dialog)  Indices=[4]  OutputSizes=1
  Selector{4,8..9,13} (4 alike) : Selector  IndexMode=Zero-based  InputPortWidth=6  IndexOptions=Index vector (dialog)  Indices=[2]  OutputSizes=1
  Switch{1..3,6} (4 alike) : Switch  Criteria=u2 ~= 0  RndMeth=Zero  InputSameDT=on
      settings: AttributesFormatString=Criteria=%<Criteria>
  UnitDelay : UnitDelay  InitialCondition=TYP_EXT_LIGHTS.CSW_OFF_EL  SampleTime=-1
      settings: AttributesFormatString=IC = %<X0>
  R_EXT_LIGHTS_WORLD_WITHOUT_ALS : Outport  OutDataTypeStr=Enum: TYP_EXT_LIGHTS  OutputWhenDisabled=reset  InitialOutput=TYP_EXT_LIGHTS.CSW_OFF_EL
      settings: AttributesFormatString=Type : %<OutDataTypeStr>\nInit :%<InitialOutput>
  wires:
  CSW_LINE_2/1 -> [CSW_LINE_2]
  INIT/1 -> [INIT]
  VEHICLE_STATE/1 -> [VEHICLE_STATE]
  CSW_LINE_4/1 -> [CSW_LINE_4]
  Switch2/1 -> Switch1/3
  UnitDelay/1 -> Switch2/3
  Constant5/1 -> Switch2/1
  LogicalOperator5/1 -> Switch2/2
  [CSW_LINE_4] -> Selector7/1
  [CSW_LINE_2] -> Selector6/1
  [CSW_LINE_2] -> Selector4/1
  Switch1/1 -> Switch3/3
  [R_EXT_LIGHTS_WORLD_WITHOUT_ALS] -> UnitDelay/1
  Constant3/1 -> Switch6/1
  Switch3/1 -> Switch6/3
  Selector4/1 -> RSA_DetectIncrease_v01_3/1
  Constant1/1 -> Switch1/1
  Constant4/1 -> Switch3/1
  Switch6/1 -> [R_EXT_LIGHTS_WORLD_WITHOUT_ALS]
  [INIT] -> Switch6/2
  [R_EXT_LIGHTS_WORLD_WITHOUT_ALS] -> R_EXT_LIGHTS_WORLD_WITHOUT_ALS/1
  RSA_DetectIncrease_v01_3/1 -> Switch3/2
  RSA_DetectIncrease_v01_1/1 -> Switch1/2
  Constant7/1 -> RelationalOperator3/2
  [VEHICLE_STATE] -> RelationalOperator3/1
  RelationalOperator3/1 -> RSA_DetectIncrease_v01_4/1
  LogicalOperator6/1 -> LogicalOperator7/2
  RSA_DetectIncrease_v01_4/1 -> LogicalOperator7/1
  [CSW_LINE_2] -> Selector1/1
  [CSW_LINE_4] -> Selector5/1
  [CSW_LINE_2] -> Selector8/1
  Selector8/1 -> LogicalOperator11/1
  Selector5/1 -> LogicalOperator15/1
  Selector1/1 -> LogicalOperator14/1
  LogicalOperator7/1 -> LogicalOperator5/2
  [CSW_LINE_2] -> Selector9/1
  LogicalOperator9/1 -> RSA_DetectIncrease_v01_1/1
  Selector9/1 -> LogicalOperator8/1
  LogicalOperator8/1 -> LogicalOperator9/2
  Selector6/1 -> LogicalOperator9/1
  [CSW_LINE_2] -> Selector12/1
  [CSW_LINE_2] -> Selector13/1
  Selector13/1 -> LogicalOperator12/1
  Selector12/1 -> LogicalOperator13/1
  Selector7/1 -> LogicalOperator10/1
  LogicalOperator13/1 -> LogicalOperator10/2
  LogicalOperator12/1 -> LogicalOperator10/3
  LogicalOperator10/1 -> LogicalOperator5/1
  LogicalOperator11/1 -> LogicalOperator6/1
  LogicalOperator14/1 -> LogicalOperator6/2
  LogicalOperator15/1 -> LogicalOperator6/3

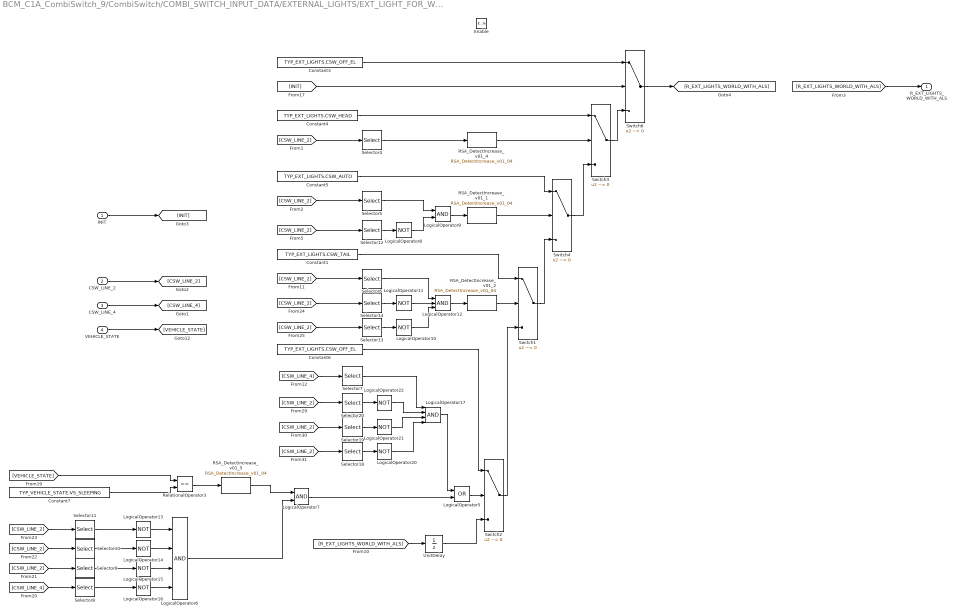
== system BCM_C1A_CombiSwitch_9/CombiSwitch/COMBI_SWITCH_INPUT_DATA/EXTERNAL_LIGHTS/EXT_LIGHT_FOR_WORLD_WITH_ALS ==
  INIT : Inport  OutDataTypeStr=boolean
      settings: AttributesFormatString=Type : %<OutDataTypeStr>
  CSW_LINE_2 : Inport  Port=2  OutDataTypeStr=boolean  PortDimensions=6
      settings: AttributesFormatString=Type : %<OutDataTypeStr>
  CSW_LINE_4 : Inport  Port=3  OutDataTypeStr=boolean  PortDimensions=6
      settings: AttributesFormatString=Type : %<OutDataTypeStr>
  VEHICLE_STATE : Inport  Port=4  OutDataTypeStr=Enum: TYP_VEHICLE_STATE
      settings: AttributesFormatString=Type : %<OutDataTypeStr>
  Enable : EnablePort  StatesWhenEnabling=reset
      settings: AttributesFormatString=State : %<StatesWhenEnabling>
  Constant1 : Constant  Value=TYP_EXT_LIGHTS.CSW_TAIL  OutDataTypeStr=Enum: TYP_EXT_LIGHTS  SampleTime=-1
  Constant3 : Constant  Value=TYP_EXT_LIGHTS.CSW_OFF_EL  OutDataTypeStr=Enum: TYP_EXT_LIGHTS  SampleTime=-1
  Constant4 : Constant  Value=TYP_EXT_LIGHTS.CSW_HEAD  OutDataTypeStr=Enum: TYP_EXT_LIGHTS  SampleTime=-1
  Constant5 : Constant  Value=TYP_EXT_LIGHTS.CSW_AUTO  OutDataTypeStr=Enum: TYP_EXT_LIGHTS  SampleTime=-1
  Constant6 : Constant  Value=TYP_EXT_LIGHTS.CSW_OFF_EL  OutDataTypeStr=Enum: TYP_EXT_LIGHTS  SampleTime=-1
  Constant7 : Constant  Value=TYP_VEHICLE_STATE.VS_SLEEPING  OutDataTypeStr=Enum: TYP_VEHICLE_STATE  SampleTime=-1
  LogicalOperator{8,10..11,13..16,20..22} (10 alike) : Logic  Operator=NOT  OutDataTypeStr=boolean
  LogicalOperator12 : Logic  Inputs=3  OutDataTypeStr=boolean
  LogicalOperator17 : Logic  Inputs=4  OutDataTypeStr=boolean
  LogicalOperator5 : Logic  Operator=OR  OutDataTypeStr=boolean
  LogicalOperator6 : Logic  Inputs=4  OutDataTypeStr=boolean
  LogicalOperator7 : Logic  OutDataTypeStr=boolean
  LogicalOperator9 : Logic  OutDataTypeStr=boolean
  RSA_DetectIncrease_v01_{1..2,4..5} (4 alike) : Renault_Library/Complex blocks/Logic & Bit Operations/RSA_DetectIncrease_v01_04  Tag=[LIB]  chkini=off  vinit=false
      settings: AttributesFormatString=%<MaskType> : Ver : 01.04\nCompare the Input with Initial Value = %<chkini>\nInitial Value : = %<vinit>
  RelationalOperator3 : RelationalOperator  Operator===  OutDataTypeStr=boolean  RndMeth=Nearest  InputSameDT=on
  Selector{5,10,14,19} (4 alike) : Selector  IndexMode=Zero-based  InputPortWidth=6  IndexOptions=Index vector (dialog)  Indices=[3]  OutputSizes=1
  Selector{4,11..13,18} (5 alike) : Selector  IndexMode=Zero-based  InputPortWidth=6  IndexOptions=Index vector (dialog)  Indices=[2]  OutputSizes=1
  Selector{6..9,20} (5 alike) : Selector  IndexMode=Zero-based  InputPortWidth=6  IndexOptions=Index vector (dialog)  Indices=[4]  OutputSizes=1
  Switch{1..4,6} (5 alike) : Switch  Criteria=u2 ~= 0  RndMeth=Zero  InputSameDT=on
      settings: AttributesFormatString=Criteria=%<Criteria>
  UnitDelay : UnitDelay  InitialCondition=TYP_EXT_LIGHTS.CSW_OFF_EL  SampleTime=-1
      settings: AttributesFormatString=IC = %<X0>
  R_EXT_LIGHTS_WORLD_WITH_ALS : Outport  OutDataTypeStr=Enum: TYP_EXT_LIGHTS  OutputWhenDisabled=reset  InitialOutput=TYP_EXT_LIGHTS.CSW_OFF_EL
      settings: AttributesFormatString=Type : %<OutDataTypeStr>\nInit :%<InitialOutput>
  wires:
  CSW_LINE_4/1 -> [CSW_LINE_4]
  VEHICLE_STATE/1 -> [VEHICLE_STATE]
  INIT/1 -> [INIT]
  CSW_LINE_2/1 -> [CSW_LINE_2]
  [INIT] -> Switch6/2
  Switch6/1 -> [R_EXT_LIGHTS_WORLD_WITH_ALS]
  Constant5/1 -> Switch4/1
  Constant4/1 -> Switch3/1
  Constant1/1 -> Switch1/1
  Selector4/1 -> RSA_DetectIncrease_v01_4/1
  Switch3/1 -> Switch6/3
  Constant3/1 -> Switch6/1
  [R_EXT_LIGHTS_WORLD_WITH_ALS] -> UnitDelay/1
  Switch4/1 -> Switch3/3
  Switch1/1 -> Switch4/3
  [CSW_LINE_2] -> Selector4/1
  [CSW_LINE_2] -> Selector5/1
  [CSW_LINE_2] -> Selector6/1
  [CSW_LINE_4] -> Selector7/1
  LogicalOperator5/1 -> Switch2/2
  Constant6/1 -> Switch2/1
  UnitDelay/1 -> Switch2/3
  Switch2/1 -> Switch1/3
  [R_EXT_LIGHTS_WORLD_WITH_ALS] -> R_EXT_LIGHTS_WORLD_WITH_ALS/1
  Constant7/1 -> RelationalOperator3/2
  [VEHICLE_STATE] -> RelationalOperator3/1
  RelationalOperator3/1 -> RSA_DetectIncrease_v01_5/1
  LogicalOperator6/1 -> LogicalOperator7/2
  RSA_DetectIncrease_v01_5/1 -> LogicalOperator7/1
  [CSW_LINE_4] -> Selector8/1
  [CSW_LINE_2] -> Selector9/1
  [CSW_LINE_2] -> Selector10/1
  [CSW_LINE_2] -> Selector11/1
  Selector10/1 -> LogicalOperator14/1
  Selector9/1 -> LogicalOperator15/1
  Selector11/1 -> LogicalOperator13/1
  Selector8/1 -> LogicalOperator16/1
  LogicalOperator7/1 -> LogicalOperator5/2
  RSA_DetectIncrease_v01_4/1 -> Switch3/2
  RSA_DetectIncrease_v01_1/1 -> Switch4/2
  RSA_DetectIncrease_v01_2/1 -> Switch1/2
  [CSW_LINE_2] -> Selector12/1
  Selector5/1 -> LogicalOperator9/1
  Selector12/1 -> LogicalOperator8/1
  LogicalOperator8/1 -> LogicalOperator9/2
  LogicalOperator9/1 -> RSA_DetectIncrease_v01_1/1
  [CSW_LINE_2] -> Selector14/1
  [CSW_LINE_2] -> Selector13/1
  Selector14/1 -> LogicalOperator11/1
  Selector13/1 -> LogicalOperator10/1
  LogicalOperator11/1 -> LogicalOperator12/2
  LogicalOperator12/1 -> RSA_DetectIncrease_v01_2/1
  LogicalOperator10/1 -> LogicalOperator12/3
  Selector6/1 -> LogicalOperator12/1
  LogicalOperator13/1 -> LogicalOperator6/1
  LogicalOperator14/1 -> LogicalOperator6/2
  LogicalOperator15/1 -> LogicalOperator6/3
  LogicalOperator16/1 -> LogicalOperator6/4
  [CSW_LINE_2] -> Selector20/1
  [CSW_LINE_2] -> Selector19/1
  [CSW_LINE_2] -> Selector18/1
  Selector19/1 -> LogicalOperator21/1
  Selector18/1 -> LogicalOperator20/1
  Selector20/1 -> LogicalOperator22/1
  Selector7/1 -> LogicalOperator17/1
  LogicalOperator22/1 -> LogicalOperator17/2
  LogicalOperator21/1 -> LogicalOperator17/3
  LogicalOperator20/1 -> LogicalOperator17/4
  LogicalOperator17/1 -> LogicalOperator5/1

== stateflow chart BCM_C1A_CombiSwitch_9/CombiSwitch/CSW_FAILURE_DETECTION/CSW_FAILURE_DETECTION_FCT ==
  state CSW_FAILURE_DETECTION
    state NO_CSW_FAILURE_DETECTION_TEST
    state CSW_FAILURE_DETECTION_TEST
      state NO_CSW_FAILURE_CONFIRMATION
        state NO_CSW_FAILURE
          entry:
          COMBI_SW_FAILURE_TFAIL=false;
          COMBI_SW_FAILURE_TCONF=false;
          CSW_IN_FAILURE_MODE=false;
        state WAITING_CSW_FAILURE_COME_BACK_IN_NORMAL
        state WAITING_CSW_FAILURE_CONFIRMATION
          entry:
          COMBI_SW_FAILURE_TFAIL=true;
        (default) -> NO_CSW_FAILURE
        NO_CSW_FAILURE -> WAITING_CSW_FAILURE_CONFIRMATION : [COMBI_SW_FAILURE]
        WAITING_CSW_FAILURE_CONFIRMATION -> NO_CSW_FAILURE [order 1] : [!COMBI_SW_FAILURE ...
            | && !COMBI_SW_FAILURE_TCONF]
        WAITING_CSW_FAILURE_COME_BACK_IN_NORMAL -> NO_CSW_FAILURE [order 2] : after(COMBI_SW_FAILURE_DETECTED_TM,tick)
        WAITING_CSW_FAILURE_COME_BACK_IN_NORMAL -> WAITING_CSW_FAILURE_CONFIRMATION [order 1] : [COMBI_SW_FAILURE]
        WAITING_CSW_FAILURE_CONFIRMATION -> WAITING_CSW_FAILURE_COME_BACK_IN_NORMAL [order 2] : [!COMBI_SW_FAILURE ...
            | && COMBI_SW_FAILURE_TCONF]
      state CSW_FAILURE_CONFIRMATION
        entry:
        COMBI_SW_FAILURE_TFAIL=true;
        COMBI_SW_FAILURE_TCONF=true;
        CSW_IN_FAILURE_MODE=true;
      (junction 38) -> NO_CSW_FAILURE_CONFIRMATION [order 2]
      CSW_FAILURE_CONFIRMATION -> WAITING_CSW_FAILURE_COME_BACK_IN_NORMAL : [!COMBI_SW_FAILURE]
      (default) -> (junction 38)
      (junction 38) -> CSW_FAILURE_CONFIRMATION [order 1] : [COMBI_SW_FAILURE_TCONF==true ...
          | && COMBI_SW_FAILURE==true]
      WAITING_CSW_FAILURE_CONFIRMATION -> CSW_FAILURE_CONFIRMATION [order 3] : after(COMBI_SW_FAILURE_DETECTED_TM,tick)
    (junction 18) -> NO_CSW_FAILURE_DETECTION_TEST [order 2]
    NO_CSW_FAILURE_DETECTION_TEST -> CSW_FAILURE_DETECTION_TEST : [IN_DRIVING_CYCLE]
    CSW_FAILURE_DETECTION_TEST -> NO_CSW_FAILURE_DETECTION_TEST : [!IN_DRIVING_CYCLE]
    (default) -> (junction 18)
    (junction 18) -> CSW_FAILURE_DETECTION_TEST [order 1] : [IN_DRIVING_CYCLE]
  (default) -> CSW_FAILURE_DETECTION : {
      | COMBI_SW_FAILURE_TFAIL=false;
      | COMBI_SW_FAILURE_TCONF=false;
      | CSW_IN_FAILURE_MODE=false;
      | }
  CSW_FAILURE_DETECTION -> CSW_FAILURE_DETECTION : [hasChangedFrom(RAZ_BY_DIAG,true)]
      | {
      | COMBI_SW_FAILURE_TFAIL=false;
      | COMBI_SW_FAILURE_TCONF=false;
      | CSW_IN_FAILURE_MODE=false;
      | }
  data: COMBI_SW_FAILURE_TFAIL output boolean; IN_DRIVING_CYCLE input boolean; RAZ_BY_DIAG input boolean; COMBI_SW_FAILURE input boolean; COMBI_SW_FAILURE_DETECTED_TM input uint16; COMBI_SW_FAILURE_TCONF output boolean; CSW_IN_FAILURE_MODE output boolean

== stateflow chart BCM_C1A_CombiSwitch_9/CombiSwitch/LIGHTING_FAILURE_DETECTION/LIGHTING_FAILURE_DETECTION_FCT ==
  state LIGHTING_FAILURE_DETECTION
    state NO_LIGHTING_FAILURE_DETECTION_TEST
    state LIGHTING_FAILURE_DETECTION_TEST
      state NO_LIGHTING_FAILURE_CONFIRMATION
        state NO_LIGHTING_FAILURE
          entry:
          COMBI_SW_LIGHTING_FAILURE_TFAIL=false;
          COMBI_SW_LIGHTING_FAILURE_TCONF=false;
          LIGHTING_CSW_FAILURE_MODE=false;
        state WAITING_CSW_FAILURE_COME_BACK_IN_NORMAL
        state WAITING_LIGHTING_FAILURE_CONFIRMATION
        (default) -> NO_LIGHTING_FAILURE
        NO_LIGHTING_FAILURE -> WAITING_LIGHTING_FAILURE_CONFIRMATION : [COMBI_SW_LIGHTING_FAILURE]
        WAITING_LIGHTING_FAILURE_CONFIRMATION -> NO_LIGHTING_FAILURE [order 1] : [!COMBI_SW_LIGHTING_FAILURE ...
            | && !COMBI_SW_LIGHTING_FAILURE_TCONF]
        WAITING_CSW_FAILURE_COME_BACK_IN_NORMAL -> NO_LIGHTING_FAILURE [order 2] : after(COMBI_SW_FAILURE_DETECTED_TM,tick)
        WAITING_LIGHTING_FAILURE_CONFIRMATION -> WAITING_CSW_FAILURE_COME_BACK_IN_NORMAL [order 3] : [!COMBI_SW_LIGHTING_FAILURE ...
            | && COMBI_SW_LIGHTING_FAILURE_TCONF]
        WAITING_CSW_FAILURE_COME_BACK_IN_NORMAL -> WAITING_LIGHTING_FAILURE_CONFIRMATION [order 1] : [COMBI_SW_LIGHTING_FAILURE]
      state LIGHTING_FAILURE_CONFIRMATION
        entry:
        COMBI_SW_LIGHTING_FAILURE_TFAIL=true;
        COMBI_SW_LIGHTING_FAILURE_TCONF=true;
        LIGHTING_CSW_FAILURE_MODE=true;
      (junction 42) -> NO_LIGHTING_FAILURE_CONFIRMATION [order 2]
      LIGHTING_FAILURE_CONFIRMATION -> WAITING_CSW_FAILURE_COME_BACK_IN_NORMAL : [!COMBI_SW_LIGHTING_FAILURE]
      (default) -> (junction 42)
      (junction 42) -> LIGHTING_FAILURE_CONFIRMATION [order 1] : [COMBI_SW_LIGHTING_FAILURE_TCONF==true ...
          | && COMBI_SW_LIGHTING_FAILURE==true]
      WAITING_LIGHTING_FAILURE_CONFIRMATION -> LIGHTING_FAILURE_CONFIRMATION [order 2] : after(COMBI_SW_FAILURE_DETECTED_TM,tick)
    (junction 18) -> NO_LIGHTING_FAILURE_DETECTION_TEST [order 2]
    NO_LIGHTING_FAILURE_DETECTION_TEST -> LIGHTING_FAILURE_DETECTION_TEST : [IN_DRIVING_CYCLE]
    LIGHTING_FAILURE_DETECTION_TEST -> NO_LIGHTING_FAILURE_DETECTION_TEST : [!IN_DRIVING_CYCLE]
    (default) -> (junction 18)
    (junction 18) -> LIGHTING_FAILURE_DETECTION_TEST [order 1] : [IN_DRIVING_CYCLE]
  (default) -> LIGHTING_FAILURE_DETECTION : {
      | COMBI_SW_LIGHTING_FAILURE_TFAIL=false;
      | COMBI_SW_LIGHTING_FAILURE_TCONF=false;
      | LIGHTING_CSW_FAILURE_MODE=false;
      | }
  LIGHTING_FAILURE_DETECTION -> LIGHTING_FAILURE_DETECTION : [hasChangedFrom(RAZ_BY_DIAG,true)]
      | {
      | COMBI_SW_LIGHTING_FAILURE_TFAIL=false;
      | COMBI_SW_LIGHTING_FAILURE_TCONF=false;
      | LIGHTING_CSW_FAILURE_MODE=false;
      | }
  data: IN_DRIVING_CYCLE input boolean; RAZ_BY_DIAG input boolean; COMBI_SW_LIGHTING_FAILURE input boolean; COMBI_SW_FAILURE_DETECTED_TM input uint16; COMBI_SW_LIGHTING_FAILURE_TFAIL output boolean; COMBI_SW_LIGHTING_FAILURE_TCONF output boolean; LIGHTING_CSW_FAILURE_MODE output boolean
